simulink model "Zad3"  (R2020b)
settings: Solver=VariableStepAuto  StartTime=0.0  StopTime=0.0  RelTol=1e-3
undefined symbols (not defined in the file): H, W
libraries: CPOiS_SourcesSinks x5, CPOiS_LinearTransforms x2, CPOiS_General x1, simulink_extras x1, CPOiS_DataManipulation x1, CPOiS_DataManipulation_DataTypeConversion x1
settings Model: Creator=Krystian  LastModifiedBy=Krystian

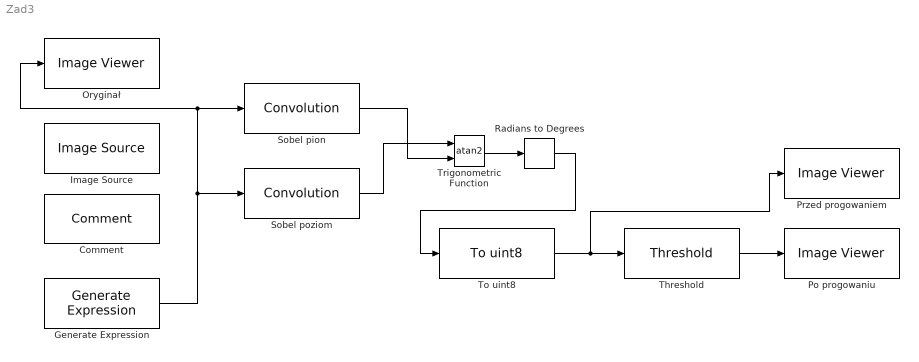
== system Zad3 ==
  Comment : CPOiS_General/Comment
      settings: SourceProductName=CPOiS - Digital image and signal processing
  Generate Expression : CPOiS_SourcesSinks/Generate Expression  Width=256  Height=256  Expression=(W-128).^2+(H-128).^2-50^2
      settings: SourceProductName=CPOiS - Digital image and signal processing
  Image Source : CPOiS_SourcesSinks/Image Source  FileSelection=eight.tif
      settings: SourceProductName=CPOiS - Digital image and signal processing
  Oryginał : CPOiS_SourcesSinks/Image Viewer
      settings: SourceProductName=CPOiS - Digital image and signal processing
  Po progowaniu : CPOiS_SourcesSinks/Image Viewer
      settings: SourceProductName=CPOiS - Digital image and signal processing
  Przed progowaniem : CPOiS_SourcesSinks/Image Viewer
      settings: SourceProductName=CPOiS - Digital image and signal processing
  Radians to Degrees : simulink_extras/Transformations/Radians to Degrees
  Sobel pion : CPOiS_LinearTransforms/Convolution  ConvolutionMatrix=[-1,0,1;-2,0,2;-1,0,1]
      settings: SourceProductName=CPOiS - Digital image and signal processing
  Sobel poziom : CPOiS_LinearTransforms/Convolution  ConvolutionMatrix=[-1,-2,-1;0,0,0;1,2,1]
      settings: SourceProductName=CPOiS - Digital image and signal processing
  Threshold : CPOiS_DataManipulation/Threshold  Threshold=127
      settings: SourceProductName=CPOiS - Digital image and signal processing
  To uint8 : CPOiS_DataManipulation_DataTypeConversion/To uint8
      settings: SourceProductName=CPOiS - Digital image and signal processing
  Trigonometric Function : Trigonometry  Operator=atan2
  wires:
  Threshold/1 -> Po progowaniu/1
  Trigonometric Function/1 -> Radians to Degrees/1
  To uint8/1 -> Threshold/1, Przed progowaniem/1
  Radians to Degrees/1 -> To uint8/1
  Sobel pion/1 -> Trigonometric Function/2
  Sobel poziom/1 -> Trigonometric Function/1
  Generate Expression/1 -> Sobel poziom/1, Oryginał/1, Sobel pion/1
